simulink model "DirectedEvent3_2018a"  (R2018a)
settings: Solver=VariableStepAuto  StartTime=0.0  StopTime=0.1  RelTol=1e-3
settings Model: Creator=86188  LastModifiedBy=apple

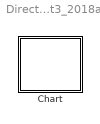
== system DirectedEvent3_2018a ==
  Chart : Stateflow chart  TreatAsAtomicUnit=on

== stateflow chart DirectedEvent3_2018a/Chart ==
  state AM
    state A [parallel]
      settings: executionOrder=1
      state A1
        en: fprintf("en_A1")
        ex: fprintf("ex_A1")
      state A2
        en: fprintf("en_A2")
        ex: fprintf("ex_A2")
      (default) -> A1
      A1 -> A2 : [data==1]{send(E_one,AM.B)}
      A2 -> A1 : E_two
    state B [parallel]
      settings: executionOrder=2
      state B1
        en: fprintf("en_B1")
        ex: fprintf("ex_B1")
      state B2
        en: fprintf("en_B2")
        ex: fprintf("ex_B2")
      (default) -> B1
      B1 -> B2 : E_one
      B2 -> B1 : E_two
  (default) -> AM
  data: data local double =1
  events: E_one local FUNCTION_CALL_EVENT; E_two local FUNCTION_CALL_EVENT
